simulink model "MCU_FaultDiag"  (R2022b)
settings: Solver=FixedStepDiscrete  StartTime=0.0  StopTime=10.0  FixedStep=1e-4  RelTol=1e-3
values from neighbouring files (symbols this model uses):
  C_Fault_CANFaultAnalogCount_u16 = 0.0    [MCU_FaultDiag_Datadictionary.sldd]    (also in MCU_FaultDiag_Datadictionary_objects.m = myPackage.Parameter)
  C_Fault_CANFaultCoeff_f32 = 0.0    [MCU_FaultDiag_Datadictionary.sldd]    (also in MCU_FaultDiag_Datadictionary_objects.m = myPackage.Parameter)
  C_Fault_CANFaultDiagEn_u8 = 0.0    [MCU_FaultDiag_Datadictionary.sldd]    (also in MCU_FaultDiag_Datadictionary_objects.m = myPackage.Parameter)
  C_Fault_CANFaultErrCode_u16 = 0.0    [MCU_FaultDiag_Datadictionary.sldd]    (also in MCU_FaultDiag_Datadictionary_objects.m = myPackage.Parameter)
  C_Fault_CANFaultLevel_u8 = 0.0    [MCU_FaultDiag_Datadictionary.sldd]    (also in MCU_FaultDiag_Datadictionary_objects.m = myPackage.Parameter)
  C_Fault_CANFaultTestbedCount_u16 = 0.0    [MCU_FaultDiag_Datadictionary.sldd]    (also in MCU_FaultDiag_Datadictionary_objects.m = myPackage.Parameter)
  C_Fault_CANFaultVehicleCount_u16 = 0.0    [MCU_FaultDiag_Datadictionary.sldd]    (also in MCU_FaultDiag_Datadictionary_objects.m = myPackage.Parameter)
  C_Fault_IaCircuitConfirmCnt_u16 = 0.0    [MCU_FaultDiag_Datadictionary.sldd]    (also in MCU_FaultDiag_Datadictionary_objects.m = myPackage.Parameter)
  C_Fault_IaCircuitConfirmDownTh_u16 = 0.0    [MCU_FaultDiag_Datadictionary.sldd]    (also in MCU_FaultDiag_Datadictionary_objects.m = myPackage.Parameter)
  C_Fault_IaCircuitConfirmUpTh_u16 = 0.0    [MCU_FaultDiag_Datadictionary.sldd]    (also in MCU_FaultDiag_Datadictionary_objects.m = myPackage.Parameter)
  C_Fault_IaCircuitFaultCoeff_f32 = 0.0    [MCU_FaultDiag_Datadictionary.sldd]    (also in MCU_FaultDiag_Datadictionary_objects.m = myPackage.Parameter)
  C_Fault_IaCircuitFaultDiagEn_u8 = 0.0    [MCU_FaultDiag_Datadictionary.sldd]    (also in MCU_FaultDiag_Datadictionary_objects.m = myPackage.Parameter)
  C_Fault_IaCircuitFaultLevel_u8 = 0.0    [MCU_FaultDiag_Datadictionary.sldd]    (also in MCU_FaultDiag_Datadictionary_objects.m = myPackage.Parameter)
  C_Fault_IaConfirmCnt_u16 = 0.0    [MCU_FaultDiag_Datadictionary.sldd]    (also in MCU_FaultDiag_Datadictionary_objects.m = myPackage.Parameter; MCU_Fault_Datadictionary_objects.m = myPackage.Parameter; MCU_Fault_Datadictionary_objects.sldd)
  C_Fault_IaInstantFaultCoeff_f32 = 0.0    [MCU_FaultDiag_Datadictionary.sldd]    (also in MCU_FaultDiag_Datadictionary_objects.m = myPackage.Parameter)
  C_Fault_IaInstantFaultDiagEn_u8 = 0.0    [MCU_FaultDiag_Datadictionary.sldd]    (also in MCU_FaultDiag_Datadictionary_objects.m = myPackage.Parameter)
  C_Fault_IaInstantFaultLevel_u8 = 0.0    [MCU_FaultDiag_Datadictionary.sldd]    (also in MCU_FaultDiag_Datadictionary_objects.m = myPackage.Parameter)
  C_Fault_IaOverLoadConfirmCnt_u16 = 0.0    [MCU_FaultDiag_Datadictionary.sldd]    (also in MCU_FaultDiag_Datadictionary_objects.m = myPackage.Parameter)
  C_Fault_IaOverLoadFaultCoeff_f32 = 0.0    [MCU_FaultDiag_Datadictionary.sldd]    (also in MCU_FaultDiag_Datadictionary_objects.m = myPackage.Parameter)
  C_Fault_IaOverLoadFaultDiagEn_u8 = 0.0    [MCU_FaultDiag_Datadictionary.sldd]    (also in MCU_FaultDiag_Datadictionary_objects.m = myPackage.Parameter)
  C_Fault_IaOverLoadFaultErrCode_u16 = 0.0    [MCU_FaultDiag_Datadictionary.sldd]    (also in MCU_FaultDiag_Datadictionary_objects.m = myPackage.Parameter)
  C_Fault_IaOverLoadFaultLevel_u8 = 0.0    [MCU_FaultDiag_Datadictionary.sldd]    (also in MCU_FaultDiag_Datadictionary_objects.m = myPackage.Parameter)
  C_Fault_IbCircuitConfirmCnt_u16 = 0.0    [MCU_FaultDiag_Datadictionary.sldd]    (also in MCU_FaultDiag_Datadictionary_objects.m = myPackage.Parameter)
  C_Fault_IbCircuitConfirmDownTh_u16 = 0.0    [MCU_FaultDiag_Datadictionary.sldd]    (also in MCU_FaultDiag_Datadictionary_objects.m = myPackage.Parameter)
  C_Fault_IbCircuitConfirmUpTh_u16 = 0.0    [MCU_FaultDiag_Datadictionary.sldd]    (also in MCU_FaultDiag_Datadictionary_objects.m = myPackage.Parameter)
  C_Fault_IbCircuitFaultCoeff_f32 = 0.0    [MCU_FaultDiag_Datadictionary.sldd]    (also in MCU_FaultDiag_Datadictionary_objects.m = myPackage.Parameter)
  C_Fault_IbCircuitFaultDiagEn_u8 = 0.0    [MCU_FaultDiag_Datadictionary.sldd]    (also in MCU_FaultDiag_Datadictionary_objects.m = myPackage.Parameter)
  C_Fault_IbCircuitFaultLevel_u8 = 0.0    [MCU_FaultDiag_Datadictionary.sldd]    (also in MCU_FaultDiag_Datadictionary_objects.m = myPackage.Parameter)
  C_Fault_IbConfirmCnt_u16 = 0.0    [MCU_FaultDiag_Datadictionary.sldd]    (also in MCU_FaultDiag_Datadictionary_objects.m = myPackage.Parameter; MCU_Fault_Datadictionary_objects.m = myPackage.Parameter; MCU_Fault_Datadictionary_objects.sldd)
  C_Fault_IbInstantFaultCoeff_f32 = 0.0    [MCU_FaultDiag_Datadictionary.sldd]    (also in MCU_FaultDiag_Datadictionary_objects.m = myPackage.Parameter)
  C_Fault_IbInstantFaultDiagEn_u8 = 0.0    [MCU_FaultDiag_Datadictionary.sldd]    (also in MCU_FaultDiag_Datadictionary_objects.m = myPackage.Parameter)
  C_Fault_IbInstantFaultLevel_u8 = 0.0    [MCU_FaultDiag_Datadictionary.sldd]    (also in MCU_FaultDiag_Datadictionary_objects.m = myPackage.Parameter)
  C_Fault_IbOverLoadConfirmCnt_u16 = 0.0    [MCU_FaultDiag_Datadictionary.sldd]    (also in MCU_FaultDiag_Datadictionary_objects.m = myPackage.Parameter)
  C_Fault_IbOverLoadFaultCoeff_f32 = 0.0    [MCU_FaultDiag_Datadictionary.sldd]    (also in MCU_FaultDiag_Datadictionary_objects.m = myPackage.Parameter)
  C_Fault_IbOverLoadFaultDiagEn_u8 = 0.0    [MCU_FaultDiag_Datadictionary.sldd]    (also in MCU_FaultDiag_Datadictionary_objects.m = myPackage.Parameter)
  C_Fault_IbOverLoadFaultErrCode_u16 = 0.0    [MCU_FaultDiag_Datadictionary.sldd]    (also in MCU_FaultDiag_Datadictionary_objects.m = myPackage.Parameter)
  C_Fault_IbOverLoadFaultLevel_u8 = 0.0    [MCU_FaultDiag_Datadictionary.sldd]    (also in MCU_FaultDiag_Datadictionary_objects.m = myPackage.Parameter)
  C_Fault_IcCircuitConfirmCnt_u16 = 0.0    [MCU_FaultDiag_Datadictionary.sldd]    (also in MCU_FaultDiag_Datadictionary_objects.m = myPackage.Parameter)
  C_Fault_IcCircuitConfirmDownTh_u16 = 0.0    [MCU_FaultDiag_Datadictionary.sldd]    (also in MCU_FaultDiag_Datadictionary_objects.m = myPackage.Parameter)
  C_Fault_IcCircuitConfirmUpTh_u16 = 0.0    [MCU_FaultDiag_Datadictionary.sldd]    (also in MCU_FaultDiag_Datadictionary_objects.m = myPackage.Parameter)
  C_Fault_IcCircuitFaultCoeff_f32 = 0.0    [MCU_FaultDiag_Datadictionary.sldd]    (also in MCU_FaultDiag_Datadictionary_objects.m = myPackage.Parameter)
  C_Fault_IcCircuitFaultDiagEn_u8 = 0.0    [MCU_FaultDiag_Datadictionary.sldd]    (also in MCU_FaultDiag_Datadictionary_objects.m = myPackage.Parameter)
  C_Fault_IcCircuitFaultLevel_u8 = 0.0    [MCU_FaultDiag_Datadictionary.sldd]    (also in MCU_FaultDiag_Datadictionary_objects.m = myPackage.Parameter)
  C_Fault_IcConfirmCnt_u16 = 0.0    [MCU_FaultDiag_Datadictionary.sldd]    (also in MCU_FaultDiag_Datadictionary_objects.m = myPackage.Parameter; MCU_Fault_Datadictionary_objects.m = myPackage.Parameter; MCU_Fault_Datadictionary_objects.sldd)
  C_Fault_IcInstantFaultCoeff_f32 = 0.0    [MCU_FaultDiag_Datadictionary.sldd]    (also in MCU_FaultDiag_Datadictionary_objects.m = myPackage.Parameter)
  C_Fault_IcInstantFaultDiagEn_u8 = 0.0    [MCU_FaultDiag_Datadictionary.sldd]    (also in MCU_FaultDiag_Datadictionary_objects.m = myPackage.Parameter)
  C_Fault_IcInstantFaultLevel_u8 = 0.0    [MCU_FaultDiag_Datadictionary.sldd]    (also in MCU_FaultDiag_Datadictionary_objects.m = myPackage.Parameter)
  C_Fault_IcOverLoadConfirmCnt_u16 = 0.0    [MCU_FaultDiag_Datadictionary.sldd]    (also in MCU_FaultDiag_Datadictionary_objects.m = myPackage.Parameter)
  C_Fault_IcOverLoadFaultCoeff_f32 = 0.0    [MCU_FaultDiag_Datadictionary.sldd]    (also in MCU_FaultDiag_Datadictionary_objects.m = myPackage.Parameter)
  C_Fault_IcOverLoadFaultDiagEn_u8 = 0.0    [MCU_FaultDiag_Datadictionary.sldd]    (also in MCU_FaultDiag_Datadictionary_objects.m = myPackage.Parameter)
  C_Fault_IcOverLoadFaultErrCode_u16 = 0.0    [MCU_FaultDiag_Datadictionary.sldd]    (also in MCU_FaultDiag_Datadictionary_objects.m = myPackage.Parameter)
  C_Fault_IcOverLoadFaultLevel_u8 = 0.0    [MCU_FaultDiag_Datadictionary.sldd]    (also in MCU_FaultDiag_Datadictionary_objects.m = myPackage.Parameter)
  C_Fault_IdcCircuitConfirmCnt_u16 = 0.0    [MCU_FaultDiag_Datadictionary.sldd]    (also in MCU_FaultDiag_Datadictionary_objects.m = myPackage.Parameter)
  C_Fault_IdcCircuitConfirmDownTh_u16 = 0.0    [MCU_FaultDiag_Datadictionary.sldd]    (also in MCU_FaultDiag_Datadictionary_objects.m = myPackage.Parameter)
  C_Fault_IdcCircuitConfirmUpTh_u16 = 0.0    [MCU_FaultDiag_Datadictionary.sldd]    (also in MCU_FaultDiag_Datadictionary_objects.m = myPackage.Parameter)
  C_Fault_IdcCircuitFaultCoeff_f32 = 0.0    [MCU_FaultDiag_Datadictionary.sldd]    (also in MCU_FaultDiag_Datadictionary_objects.m = myPackage.Parameter)
  C_Fault_IdcCircuitFaultDiagEn_u8 = 0.0    [MCU_FaultDiag_Datadictionary.sldd]    (also in MCU_FaultDiag_Datadictionary_objects.m = myPackage.Parameter)
  C_Fault_IdcCircuitFaultLevel_u8 = 0.0    [MCU_FaultDiag_Datadictionary.sldd]    (also in MCU_FaultDiag_Datadictionary_objects.m = myPackage.Parameter)
  C_Fault_SelfCheckFaultCoeff_f32 = 0.0    [MCU_FaultDiag_Datadictionary.sldd]    (also in MCU_FaultDiag_Datadictionary_objects.m = myPackage.Parameter)
  C_Fault_SelfCheckFaultDiagEn_u8 = 0.0    [MCU_FaultDiag_Datadictionary.sldd]    (also in MCU_FaultDiag_Datadictionary_objects.m = myPackage.Parameter)
  C_Fault_SelfCheckFaultLevel_u8 = 0.0    [MCU_FaultDiag_Datadictionary.sldd]    (also in MCU_FaultDiag_Datadictionary_objects.m = myPackage.Parameter)
  C_Fault_SpeedOverConfirmCnt_u16 = 0.0    [MCU_FaultDiag_Datadictionary.sldd]    (also in MCU_FaultDiag_Datadictionary_objects.m = myPackage.Parameter)
  C_Fault_SpeedOverFaultCoeff_f32 = 0.0    [MCU_FaultDiag_Datadictionary.sldd]    (also in MCU_FaultDiag_Datadictionary_objects.m = myPackage.Parameter)
  C_Fault_SpeedOverFaultDiagEn_u8 = 0.0    [MCU_FaultDiag_Datadictionary.sldd]    (also in MCU_FaultDiag_Datadictionary_objects.m = myPackage.Parameter)
  C_Fault_SpeedOverFaultLevel_u8 = 0.0    [MCU_FaultDiag_Datadictionary.sldd]    (also in MCU_FaultDiag_Datadictionary_objects.m = myPackage.Parameter)
  C_Fault_SpeedOverWarnConfirmCnt_u16 = 0.0    [MCU_FaultDiag_Datadictionary.sldd]    (also in MCU_FaultDiag_Datadictionary_objects.m = myPackage.Parameter)
  C_Fault_SpeedOverWarnFaultCoeff_f32 = 0.0    [MCU_FaultDiag_Datadictionary.sldd]    (also in MCU_FaultDiag_Datadictionary_objects.m = myPackage.Parameter)
  C_Fault_SpeedOverWarnFaultDiagEn_u8 = 0.0    [MCU_FaultDiag_Datadictionary.sldd]    (also in MCU_FaultDiag_Datadictionary_objects.m = myPackage.Parameter)
  C_Fault_SpeedOverWarnFaultLevel_u8 = 0.0    [MCU_FaultDiag_Datadictionary.sldd]    (also in MCU_FaultDiag_Datadictionary_objects.m = myPackage.Parameter)
  C_Fault_TigbtCircuitConfirmCnt_u16 = 0.0    [MCU_FaultDiag_Datadictionary.sldd]    (also in MCU_FaultDiag_Datadictionary_objects.m = myPackage.Parameter)
  C_Fault_TigbtCircuitConfirmTh_u16 = 0.0    [MCU_FaultDiag_Datadictionary.sldd]    (also in MCU_FaultDiag_Datadictionary_objects.m = myPackage.Parameter)
  C_Fault_TigbtCircuitFaultCoeff_f32 = 0.0    [MCU_FaultDiag_Datadictionary.sldd]    (also in MCU_FaultDiag_Datadictionary_objects.m = myPackage.Parameter)
  C_Fault_TigbtCircuitFaultDiagEn_u8 = 0.0    [MCU_FaultDiag_Datadictionary.sldd]    (also in MCU_FaultDiag_Datadictionary_objects.m = myPackage.Parameter)
  C_Fault_TigbtCircuitFaultErrCode_u16 = 0.0    [MCU_FaultDiag_Datadictionary.sldd]    (also in MCU_FaultDiag_Datadictionary_objects.m = myPackage.Parameter)
  C_Fault_TigbtCircuitFaultLevel_u8 = 0.0    [MCU_FaultDiag_Datadictionary.sldd]    (also in MCU_FaultDiag_Datadictionary_objects.m = myPackage.Parameter)
  C_Fault_TigbtOverConfirmCnt_u16 = 0.0    [MCU_FaultDiag_Datadictionary.sldd]    (also in MCU_FaultDiag_Datadictionary_objects.m = myPackage.Parameter; MCU_Fault_Datadictionary_objects.m = myPackage.Parameter; MCU_Fault_Datadictionary_objects.sldd)
  C_Fault_TigbtOverFaultCoeff_f32 = 0.0    [MCU_FaultDiag_Datadictionary.sldd]    (also in MCU_FaultDiag_Datadictionary_objects.m = myPackage.Parameter)
  C_Fault_TigbtOverFaultDiagEn_u8 = 0.0    [MCU_FaultDiag_Datadictionary.sldd]    (also in MCU_FaultDiag_Datadictionary_objects.m = myPackage.Parameter)
  C_Fault_TigbtOverFaultLevel_u8 = 0.0    [MCU_FaultDiag_Datadictionary.sldd]    (also in MCU_FaultDiag_Datadictionary_objects.m = myPackage.Parameter)
  C_Fault_TigbtOverWarnConfirmCnt_u16 = 0.0    [MCU_FaultDiag_Datadictionary.sldd]    (also in MCU_FaultDiag_Datadictionary_objects.m = myPackage.Parameter)
  C_Fault_TigbtOverWarnFaultCoeff_f32 = 0.0    [MCU_FaultDiag_Datadictionary.sldd]    (also in MCU_FaultDiag_Datadictionary_objects.m = myPackage.Parameter)
  C_Fault_TigbtOverWarnFaultDiagEn_u8 = 0.0    [MCU_FaultDiag_Datadictionary.sldd]    (also in MCU_FaultDiag_Datadictionary_objects.m = myPackage.Parameter)
  C_Fault_TigbtOverWarnFaultLevel_u8 = 0.0    [MCU_FaultDiag_Datadictionary.sldd]    (also in MCU_FaultDiag_Datadictionary_objects.m = myPackage.Parameter)
  C_Fault_TmotorCircuitConfirmCnt_u16 = 0.0    [MCU_FaultDiag_Datadictionary.sldd]    (also in MCU_FaultDiag_Datadictionary_objects.m = myPackage.Parameter)
  C_Fault_TmotorCircuitConfirmTh_u16 = 0.0    [MCU_FaultDiag_Datadictionary.sldd]    (also in MCU_FaultDiag_Datadictionary_objects.m = myPackage.Parameter)
  C_Fault_TmotorCircuitFaultCoeff_f32 = 0.0    [MCU_FaultDiag_Datadictionary.sldd]    (also in MCU_FaultDiag_Datadictionary_objects.m = myPackage.Parameter)
  C_Fault_TmotorCircuitFaultDiagEn_u8 = 0.0    [MCU_FaultDiag_Datadictionary.sldd]    (also in MCU_FaultDiag_Datadictionary_objects.m = myPackage.Parameter)
  C_Fault_TmotorCircuitFaultErrCode_u16 = 0.0    [MCU_FaultDiag_Datadictionary.sldd]    (also in MCU_FaultDiag_Datadictionary_objects.m = myPackage.Parameter)
  C_Fault_TmotorCircuitFaultLevel_u8 = 0.0    [MCU_FaultDiag_Datadictionary.sldd]    (also in MCU_FaultDiag_Datadictionary_objects.m = myPackage.Parameter)
  C_Fault_TmotorOverConfirmCnt_u16 = 0.0    [MCU_FaultDiag_Datadictionary.sldd]    (also in MCU_FaultDiag_Datadictionary_objects.m = myPackage.Parameter; MCU_Fault_Datadictionary_objects.m = myPackage.Parameter; MCU_Fault_Datadictionary_objects.sldd)
  C_Fault_TmotorOverFaultCoeff_f32 = 0.0    [MCU_FaultDiag_Datadictionary.sldd]    (also in MCU_FaultDiag_Datadictionary_objects.m = myPackage.Parameter)
  C_Fault_TmotorOverFaultDiagEn_u8 = 0.0    [MCU_FaultDiag_Datadictionary.sldd]    (also in MCU_FaultDiag_Datadictionary_objects.m = myPackage.Parameter)
  C_Fault_TmotorOverFaultLevel_u8 = 0.0    [MCU_FaultDiag_Datadictionary.sldd]    (also in MCU_FaultDiag_Datadictionary_objects.m = myPackage.Parameter)
  C_Fault_TmotorOverWarnConfirmCnt_u16 = 0.0    [MCU_FaultDiag_Datadictionary.sldd]    (also in MCU_FaultDiag_Datadictionary_objects.m = myPackage.Parameter)
  C_Fault_TmotorOverWarnFaultCoeff_f32 = 0.0    [MCU_FaultDiag_Datadictionary.sldd]    (also in MCU_FaultDiag_Datadictionary_objects.m = myPackage.Parameter)
  C_Fault_TmotorOverWarnFaultDiagEn_u8 = 0.0    [MCU_FaultDiag_Datadictionary.sldd]    (also in MCU_FaultDiag_Datadictionary_objects.m = myPackage.Parameter)
  C_Fault_TmotorOverWarnFaultLevel_u8 = 0.0    [MCU_FaultDiag_Datadictionary.sldd]    (also in MCU_FaultDiag_Datadictionary_objects.m = myPackage.Parameter)
  C_Fault_TpcuCircuitConfirmCnt_u16 = 0.0    [MCU_FaultDiag_Datadictionary.sldd]    (also in MCU_FaultDiag_Datadictionary_objects.m = myPackage.Parameter)
  C_Fault_TpcuCircuitConfirmTh_u16 = 0.0    [MCU_FaultDiag_Datadictionary.sldd]    (also in MCU_FaultDiag_Datadictionary_objects.m = myPackage.Parameter)
  C_Fault_TpcuCircuitFaultCoeff_f32 = 0.0    [MCU_FaultDiag_Datadictionary.sldd]    (also in MCU_FaultDiag_Datadictionary_objects.m = myPackage.Parameter)
  C_Fault_TpcuCircuitFaultDiagEn_u8 = 0.0    [MCU_FaultDiag_Datadictionary.sldd]    (also in MCU_FaultDiag_Datadictionary_objects.m = myPackage.Parameter)
  C_Fault_TpcuCircuitFaultErrCode_u16 = 0.0    [MCU_FaultDiag_Datadictionary.sldd]    (also in MCU_FaultDiag_Datadictionary_objects.m = myPackage.Parameter)
  C_Fault_TpcuCircuitFaultLevel_u8 = 0.0    [MCU_FaultDiag_Datadictionary.sldd]    (also in MCU_FaultDiag_Datadictionary_objects.m = myPackage.Parameter)
  C_Fault_TZFaultCoeff_f32 = 0.0    [MCU_FaultDiag_Datadictionary.sldd]    (also in MCU_FaultDiag_Datadictionary_objects.m = myPackage.Parameter)
  C_Fault_TZFaultDiagEn_u8 = 0.0    [MCU_FaultDiag_Datadictionary.sldd]    (also in MCU_FaultDiag_Datadictionary_objects.m = myPackage.Parameter)
  C_Fault_TZFaultLevel_u8 = 0.0    [MCU_FaultDiag_Datadictionary.sldd]    (also in MCU_FaultDiag_Datadictionary_objects.m = myPackage.Parameter)
  C_Fault_UdcCircuitConfirmCnt_u16 = 0.0    [MCU_FaultDiag_Datadictionary.sldd]    (also in MCU_FaultDiag_Datadictionary_objects.m = myPackage.Parameter)
  C_Fault_UdcCircuitConfirmTh_u16 = 0.0    [MCU_FaultDiag_Datadictionary.sldd]    (also in MCU_FaultDiag_Datadictionary_objects.m = myPackage.Parameter)
  C_Fault_UdcCircuitFaultCoeff_f32 = 0.0    [MCU_FaultDiag_Datadictionary.sldd]    (also in MCU_FaultDiag_Datadictionary_objects.m = myPackage.Parameter)
  C_Fault_UdcCircuitFaultDiagEn_u8 = 0.0    [MCU_FaultDiag_Datadictionary.sldd]    (also in MCU_FaultDiag_Datadictionary_objects.m = myPackage.Parameter)
  C_Fault_UdcCircuitFaultErrCode_u16 = 0.0    [MCU_FaultDiag_Datadictionary.sldd]    (also in MCU_FaultDiag_Datadictionary_objects.m = myPackage.Parameter)
  C_Fault_UdcCircuitFaultLevel_u8 = 0.0    [MCU_FaultDiag_Datadictionary.sldd]    (also in MCU_FaultDiag_Datadictionary_objects.m = myPackage.Parameter)
  C_Fault_UdcOverConfirmCnt_u16 = 0.0    [MCU_FaultDiag_Datadictionary.sldd]    (also in MCU_FaultDiag_Datadictionary_objects.m = myPackage.Parameter)
  C_Fault_UdcOverFaultCoeff_f32 = 0.0    [MCU_FaultDiag_Datadictionary.sldd]    (also in MCU_FaultDiag_Datadictionary_objects.m = myPackage.Parameter)
  C_Fault_UdcOverFaultDiagEn_u8 = 0.0    [MCU_FaultDiag_Datadictionary.sldd]    (also in MCU_FaultDiag_Datadictionary_objects.m = myPackage.Parameter)
  C_Fault_UdcOverFaultLevel_u8 = 0.0    [MCU_FaultDiag_Datadictionary.sldd]    (also in MCU_FaultDiag_Datadictionary_objects.m = myPackage.Parameter)
  C_Fault_UdcOverWarnConfirmCnt_u16 = 0.0    [MCU_FaultDiag_Datadictionary.sldd]    (also in MCU_FaultDiag_Datadictionary_objects.m = myPackage.Parameter)
  C_Fault_UdcOverWarnFaultCoeff_f32 = 0.0    [MCU_FaultDiag_Datadictionary.sldd]    (also in MCU_FaultDiag_Datadictionary_objects.m = myPackage.Parameter)
  C_Fault_UdcOverWarnFaultDiagEn_u8 = 0.0    [MCU_FaultDiag_Datadictionary.sldd]    (also in MCU_FaultDiag_Datadictionary_objects.m = myPackage.Parameter)
  C_Fault_UdcOverWarnFaultLevel_u8 = 0.0    [MCU_FaultDiag_Datadictionary.sldd]    (also in MCU_FaultDiag_Datadictionary_objects.m = myPackage.Parameter)
  ... (+8 more)
undefined symbols (not defined in the file or in its folder): AB_SAMPLE, ABC_SAMPLE, AC_SAMPLE, cAgeingMode, cSingleBoardMode, ParamCfg_CommandSource_u16, ParamCfg_IaValueDefault_u16, ParamCfg_IbValueDefault_u16, ParamCfg_IcValueDefault_u16, ParamCfg_IphaseLimitStart_u16, ParamCfg_MotorLimitStart_u16, ParamCfg_MotorLimitStop_u16, ParamCfg_SampleMode_u16, ParamCfg_SpeedLimitStart_u16, ParamCfg_SpeedLimitStop_u16, ParamCfg_TigbtLimitStart_u16, ParamCfg_TigbtLimitStop_u16, VEHICLE
libraries: simulink x62
(part 1 of 426)
settings Model: DataDictionary=MCU_FaultDiag_Datadictionary.sldd  Creator=ZYH  LastModifiedBy=ZYH
settings OptimizationCC: DefaultParameterBehavior=Inlined  EnhancedBackFolding=on  PassReuseOutputArgsAs=Individual arguments  OptimizeBlockOrder=speed  DifferentSizesBufferReuse=on  OptimizationCustomize=off  EfficientTunableParamExpr=on
settings DebuggingCC: ParameterTunabilityLossMsg=error
settings SFSimCC: MATLABDynamicMemAlloc=off
settings RTWCC: Description=Embedded Coder  SystemTargetFile=ert.tlc  GenCodeOnly=on  TemplateMakefile=ert_default_tmf
settings CodeAppCC: ForceParamTrailComments=on  IgnoreCustomStorageClasses=off  OperatorAnnotations=on  SimulinkDataObjDesc=on  SFDataObjDesc=on  InsertBlockDesc=on
settings ERTTargetCC: TargetLangStandard=C99 (ISO)  GenerateSampleERTMain=on  InlinedParameterPlacement=NonHierarchical  ERTCustomFileTemplate=example_file_process.tlc

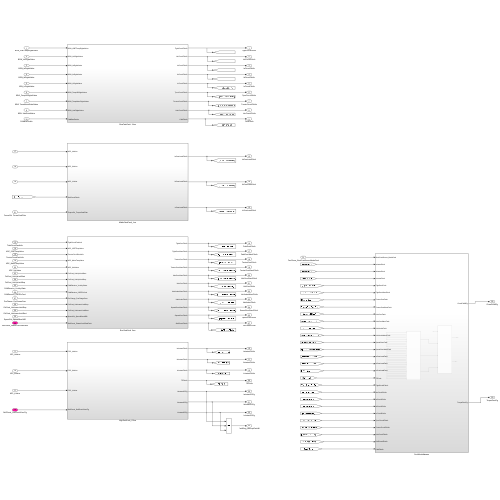
[thumbnail: Simulink's stored preview of the top-level diagram]
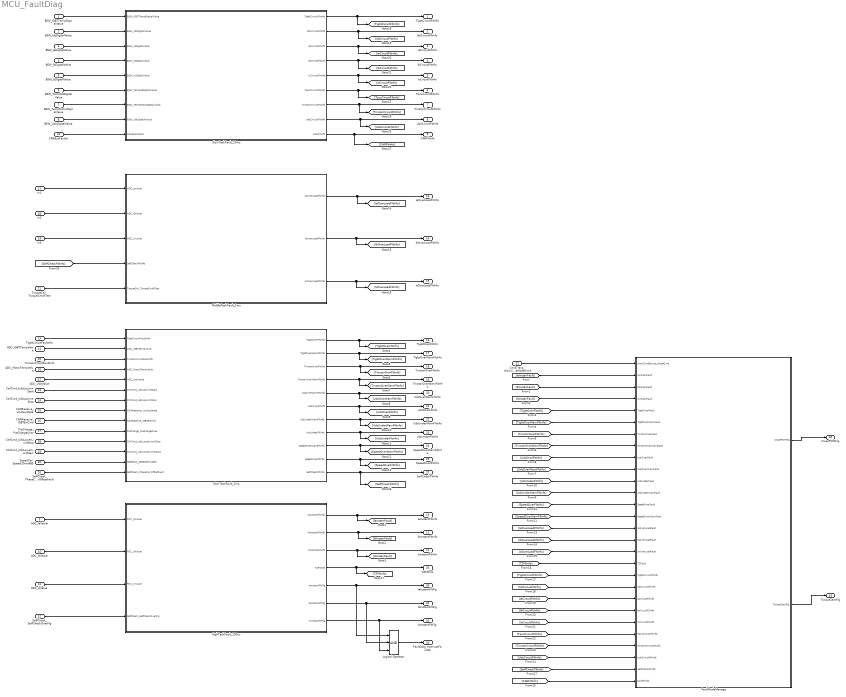
== system MCU_FaultDiag ==
  BSW_IGBTTempDigitalValue : Inport
  BSW_IdcDigitalValue : Inport  Port=2
  BSW_IaDigitalValue : Inport  Port=3
  BSW_IbDigitalValue : Inport  Port=4
  BSW_IcDigitalValue : Inport  Port=5
  BSW_TempHSDigitalValue : Inport  Port=6
  BSW_TempMotorDigitalValue : Inport  Port=7
  BSW_UdcDigitalValue : Inport  Port=8
  ADC_IaValue : Inport  Port=9
  ADC_IbValue : Inport  Port=10
  ADC_IcValue : Inport  Port=11
  SelfCheck_SelfCheckOverFlg : Inport  Port=12
  TigbtCircuitFaultInfo : Inport  Port=13  OutDataTypeStr=Bus: FaultBus
  ADC_IGBTTempValue : Inport  Port=14
  TmotorCircuitFaultInfo : Inport  Port=15  OutDataTypeStr=Bus: FaultBus
  ADC_MotorTempValue : Inport  Port=16
  In1 : Inport  Port=17
  In2 : Inport  Port=18
  In3 : Inport  Port=19
  SelfCheck_PhaseCurrOffsetFault : Inport  Port=20
  TorqueCtrl_TorqueCmdFilter : Inport  Port=21
  ADC_UdcValue : Inport  Port=22
  CtrlCmd_UdcUpLimitStart : Inport  Port=23
  CtrlCmd_UdcUpLimitStop : Inport  Port=24
  CANReceive_VcuKeyState : Inport  Port=25
  CANReceive_IGBTEnCmd : Inport  Port=26
  PreCharge_PreChargeOver : Inport  Port=27
  CtrlCmd_UdcLowerLimitStop : Inport  Port=28
  CtrlCmd_UdcLowerLimitStart : Inport  Port=29
  SpeedCal_Speed20msABS : Inport  Port=30
  CmdTrans_WorkCmdSourceModeCmd : Inport  Port=31
  CANBusFaultIn : Inport  Port=32
  FaultModeManage : Subsystem
  HighTaskFault_100us : Subsystem
  Logical Operator : Logic  Inputs=3  AllPortsSameDT=off  OutDataTypeStr=boolean
  MiddleTaskFault_1ms : Subsystem
  SlowTaskFault_10ms : Subsystem
  SlowTaskFault_2ms : Subsystem
  TigbtCircuitFltInfo : Outport
  IdcCircuitFltInfo : Outport  Port=2
  IaCircuitFltInfo : Outport  Port=3
  IbCircuitFltInfo : Outport  Port=4
  IcCircuitFltInfo : Outport  Port=5
  TpcuCircuitFltInfo : Outport  Port=6
  TmotorCircuitFltInfo : Outport  Port=7
  UdcCircuitFltInfo : Outport  Port=8
  CANFltInfo : Outport  Port=9
  IaInstantFltInfo : Outport  Port=10
  IbInstantFltInfo : Outport  Port=11
  IcInstantFltInfo : Outport  Port=12
  IaOverLoadFltInfo : Outport  Port=13
  IbOverLoadFltInfo : Outport  Port=14
  IcOverLoadFltInfo : Outport  Port=15
  TigbtOverFltInfo : Outport  Port=16
  TigbtOverWarnFltInfo : Outport  Port=17
  TmotorOverFltInfo : Outport  Port=18
  TmotorOverWarnFltInfo : Outport  Port=19
  UdcOverWarnFltInfo : Outport  Port=20
  UdcOverFltInfo : Outport  Port=21
  UdcUnderWarnFltInfo : Outport  Port=22
  UdcUnderFltInfo : Outport  Port=23
  SpeedOverWarnFltInfo : Outport  Port=24
  SpeedOverFltInfo : Outport  Port=25
  TZFltInfo : Outport  Port=26
  SelfCheckFltInfo : Outport  Port=27
  ClosePWMFlg : Outport  Port=28
  TorqueZeroFlg : Outport  Port=29
  IaInstantFltFlg : Outport  Port=30
  IbInstantFltFlg : Outport  Port=31
  IcInstantFltFlg : Outport  Port=32
  FaultDiag_InterruptFaultAll : Outport  Port=33
  wires:
  ADC_IaValue/1 -> HighTaskFault_100us/1(FOC_IaValue)
  ADC_IbValue/1 -> HighTaskFault_100us/2(FOC_IbValue)
  ADC_IcValue/1 -> HighTaskFault_100us/3(FOC_IcValue)
  BSW_IGBTTempDigitalValue/1 -> SlowTaskFault_10ms/1(BSW_IGBTTempDigitalValue)
  SlowTaskFault_10ms/1(TigbtCircuitFltInfo) -> [TigbtCircuitFltInfo], TigbtCircuitFltInfo/1
  HighTaskFault_100us/1(IaInstantFltInfo) -> [IaInstanFault], IaInstantFltInfo/1
  HighTaskFault_100us/2(IbInstantFltInfo) -> [IbInstanFault], IbInstantFltInfo/1
  HighTaskFault_100us/3(IcInstantFltInfo) -> [IcInstanFault], IcInstantFltInfo/1
  BSW_IdcDigitalValue/1 -> SlowTaskFault_10ms/2(BSW_IdcDigitalValue)
  BSW_IaDigitalValue/1 -> SlowTaskFault_10ms/3(BSW_IaDigitalValue)
  BSW_IbDigitalValue/1 -> SlowTaskFault_10ms/4(BSW_IbDigitalValue)
  BSW_IcDigitalValue/1 -> SlowTaskFault_10ms/5(BSW_IcDigitalValue)
  SlowTaskFault_10ms/4(IbCircuitFltInfo) -> [IbCircuitFltInfo], IbCircuitFltInfo/1
  SlowTaskFault_10ms/3(IaCircuitFltInfo) -> [IaCircuitFltInfo], IaCircuitFltInfo/1
  SlowTaskFault_10ms/5(IcCircuitFltInfo) -> [IcCircuitFltInfo], IcCircuitFltInfo/1
  SlowTaskFault_10ms/7(TmotorCircuitFltInfo) -> [TmotorCircuitFltInfo], TmotorCircuitFltInfo/1
  SlowTaskFault_10ms/8(UdcCircuitFltInfo) -> [UdcCircuitFltInfo], UdcCircuitFltInfo/1
  BSW_TempHSDigitalValue/1 -> SlowTaskFault_10ms/6(BSW_TempHSDigitalValue)
  BSW_TempMotorDigitalValue/1 -> SlowTaskFault_10ms/7(BSW_TempMotorDigitalValue)
  BSW_UdcDigitalValue/1 -> SlowTaskFault_10ms/8(BSW_UdcDigitalValue)
  TigbtCircuitFaultInfo/1 -> SlowTaskFault_2ms/1(TigbtCircuitFaultInfo)
  TmotorCircuitFaultInfo/1 -> SlowTaskFault_2ms/3(TmotorCircuitFaultInfo)
  ADC_MotorTempValue/1 -> SlowTaskFault_2ms/4(ADC_MotorTempValue)
  ADC_IGBTTempValue/1 -> SlowTaskFault_2ms/2(ADC_IGBTTempValue)
  In1/1 -> MiddleTaskFault_1ms/1(ADC_IaValue)
  In2/1 -> MiddleTaskFault_1ms/2(ADC_IbValue)
  In3/1 -> MiddleTaskFault_1ms/3(ADC_IcValue)
  MiddleTaskFault_1ms/1(IaOverLoadFltInfo) -> IaOverLoadFltInfo/1, [IaOverLoadFltInfo]
  MiddleTaskFault_1ms/2(IbOverLoadFltInfo) -> [IbOverLoadFltInfo], IbOverLoadFltInfo/1
  MiddleTaskFault_1ms/3(IcOverLoadFltInfo) -> [IcOverLoadFltInfo], IcOverLoadFltInfo/1
  TorqueCtrl_TorqueCmdFilter/1 -> MiddleTaskFault_1ms/5(TorqueCtrl_TorqueCmdFilter)
  CtrlCmd_UdcUpLimitStop/1 -> SlowTaskFault_2ms/7(CtrlCmd_UdcUpLimitStop)
  CANReceive_VcuKeyState/1 -> SlowTaskFault_2ms/8(CANReceive_VcuKeyState)
  CANReceive_IGBTEnCmd/1 -> SlowTaskFault_2ms/9(CANReceive_IGBTEnCmd)
  PreCharge_PreChargeOver/1 -> SlowTaskFault_2ms/10(PreCharge_PreChargeOver)
  ADC_UdcValue/1 -> SlowTaskFault_2ms/5(ADC_UdcValue)
  CtrlCmd_UdcLowerLimitStop/1 -> SlowTaskFault_2ms/11(CtrlCmd_UdcLowerLimitStop)
  CtrlCmd_UdcUpLimitStart/1 -> SlowTaskFault_2ms/6(CtrlCmd_UdcUpLimitStart)
  CtrlCmd_UdcLowerLimitStart/1 -> SlowTaskFault_2ms/12(CtrlCmd_UdcLowerLimitStart)
  SpeedCal_Speed20msABS/1 -> SlowTaskFault_2ms/13(SpeedCal_Speed20msABS)
  SlowTaskFault_2ms/1(TigbtOverFltInfo) -> TigbtOverFltInfo/1, [TigbtOverFltInfo]
  SlowTaskFault_2ms/3(TmotorOverFltInfo) -> [TmotorOverFltInfo], TmotorOverFltInfo/1
  SlowTaskFault_2ms/2(TigbtOverWarnFltInfo) -> [TigbtOverWarnFltInfo], TigbtOverWarnFltInfo/1
  SlowTaskFault_2ms/4(TmotorOverWarnFltInfo) -> [TmotorOverWarnFltInfo], TmotorOverWarnFltInfo/1
  SlowTaskFault_2ms/5(UdcOverWarnFltInfo) -> [UdcOverWarnFltInfo], UdcOverWarnFltInfo/1
  SlowTaskFault_2ms/6(UdcOverFltInfo) -> [UdcOverFltInfo], UdcOverFltInfo/1
  SlowTaskFault_2ms/7(UdcUnderWarnFltInfo) -> [UdcUnderWarnFltInfo], UdcUnderWarnFltInfo/1
  SlowTaskFault_2ms/8(UdcUnderFltInfo) -> [UdcUnderFltInfo], UdcUnderFltInfo/1
  SlowTaskFault_2ms/9(SpeedOverWarnFltInfo) -> SpeedOverWarnFltInfo/1, [SpeedOverWarnFltInfo]
  SlowTaskFault_2ms/10(SpeedOverFltInfo) -> [SpeedOverFltInfo], SpeedOverFltInfo/1
  CmdTrans_WorkCmdSourceModeCmd/1 -> FaultModeManage/1(WorkCmdSource_ModeCmd)
  [IaInstanFault] -> FaultModeManage/2(IaInstanFault)
  [IbInstanFault] -> FaultModeManage/3(IbInstanFault)
  [IcInstanFault] -> FaultModeManage/4(IcInstanFault)
  [TigbtOverFltInfo] -> FaultModeManage/5(TigbtOverFault)
  [TigbtOverWarnFltInfo] -> FaultModeManage/6(TigbtOverWarnFault)
  [TmotorOverFltInfo] -> FaultModeManage/7(TmotorOverFault)
  [TmotorOverWarnFltInfo] -> FaultModeManage/8(TmotorOverWarnFault)
  [SpeedOverFltInfo] -> FaultModeManage/13(SpeedOverFault)
  [SpeedOverWarnFltInfo] -> FaultModeManage/14(SpeedOverWarnFault)
  [UdcOverFltInfo] -> FaultModeManage/9(UdcOverFault)
  [UdcOverWarnFltInfo] -> FaultModeManage/10(UdcOverWarnFault)
  [UdcUnderWarnFltInfo] -> FaultModeManage/12(UdcUnderWarnFault)
  [UdcUnderFltInfo] -> FaultModeManage/11(UdcUnderFault)
  [IaOverLoadFltInfo] -> FaultModeManage/15(IaOverLoadFault)
  [IbOverLoadFltInfo] -> FaultModeManage/16(IbOverLoadFault)
  [IcOverLoadFltInfo] -> FaultModeManage/17(IcOverLoadFault)
  HighTaskFault_100us/4(TZFltInfo) -> [TZFltInfo], TZFltInfo/1
  [TZFltInfo] -> FaultModeManage/18(TZFault)
  SlowTaskFault_10ms/2(IdcCircuitFltInfo) -> [IdcCircuitFltInfo], IdcCircuitFltInfo/1
  SlowTaskFault_10ms/6(TpcuCircuitFltInfo) -> [TpcuCircuitFltInfo], TpcuCircuitFltInfo/1
  [TpcuCircuitFltInfo] -> FaultModeManage/24(TpcuCircuitFltInfo)
  [IcCircuitFltInfo] -> FaultModeManage/23(IcCircuitFltInfo)
  [TmotorCircuitFltInfo] -> FaultModeManage/25(TmotorCircuitFltInfo)
  [IbCircuitFltInfo] -> FaultModeManage/22(IbCircuitFltInfo)
  [UdcCircuitFltInfo] -> FaultModeManage/26(UdcCircuitFltInfo)
  [IaCircuitFltInfo] -> FaultModeManage/21(IaCircuitFltInfo)
  [IdcCircuitFltInfo] -> FaultModeManage/20(IdcCircuitFltInfo)
  [TigbtCircuitFltInfo] -> FaultModeManage/19(TigbtCircuitFltInfo)
  [SelfCheckFltInfo] -> FaultModeManage/27(SelfCheckFltInfo)
  SelfCheck_SelfCheckOverFlg/1 -> HighTaskFault_100us/4(SelfCheck_SelfCheckOverFlg)
  SelfCheck_PhaseCurrOffsetFault/1 -> SlowTaskFault_2ms/14(SelfCheck_PhaseCurrOffsetFault)
  SlowTaskFault_2ms/11(SelfCheckFltInfo) -> [SelfCheckFltInfo], SelfCheckFltInfo/1
  [SelfCheckFltInfo] -> MiddleTaskFault_1ms/4(SelfCheckFltInfo)
  FaultModeManage/1(ClosePWMFlg) -> ClosePWMFlg/1
  FaultModeManage/2(TorqueZeroFlg) -> TorqueZeroFlg/1
  HighTaskFault_100us/5(IaInstantFltFlg) -> Logical Operator/1, IaInstantFltFlg/1
  HighTaskFault_100us/6(IbInstantFltFlg) -> Logical Operator/2, IbInstantFltFlg/1
  HighTaskFault_100us/7(IcInstantFltFlg) -> Logical Operator/3, IcInstantFltFlg/1
  Logical Operator/1 -> FaultDiag_InterruptFaultAll/1
  CANBusFaultIn/1 -> SlowTaskFault_10ms/9(CANBusFaultIn)
  SlowTaskFault_10ms/9(CANFltInfo) -> [CANFltInfo], CANFltInfo/1
  [CANFltInfo] -> FaultModeManage/28(CANFltInfo)

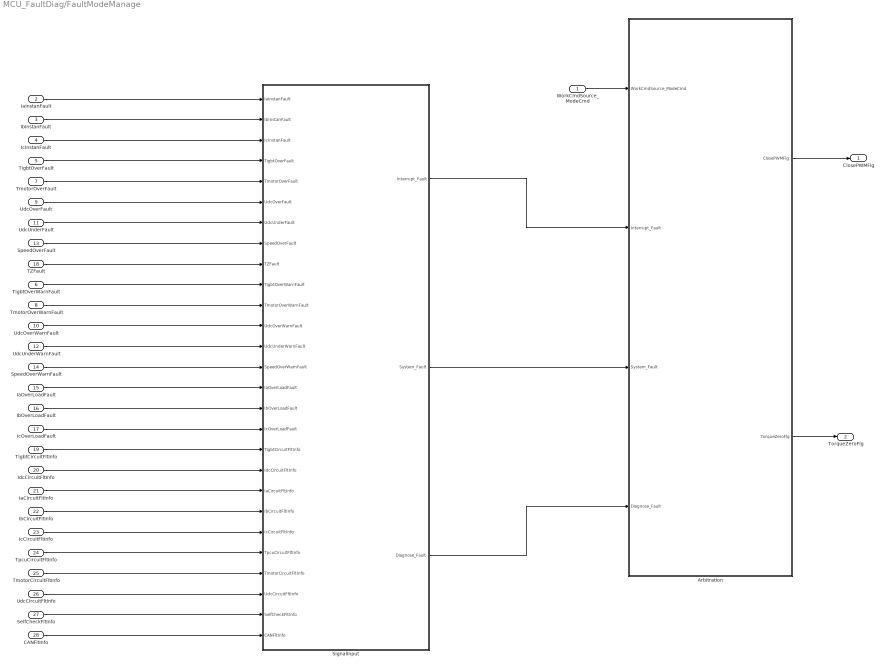
== system MCU_FaultDiag/FaultModeManage ==
  WorkCmdSource_ModeCmd : Inport
  IaInstanFault : Inport  Port=2
  IbInstanFault : Inport  Port=3
  IcInstanFault : Inport  Port=4
  TigbtOverFault : Inport  Port=5
  TigbtOverWarnFault : Inport  Port=6
  TmotorOverFault : Inport  Port=7
  TmotorOverWarnFault : Inport  Port=8
  UdcOverFault : Inport  Port=9
  UdcOverWarnFault : Inport  Port=10
  UdcUnderFault : Inport  Port=11
  UdcUnderWarnFault : Inport  Port=12
  SpeedOverFault : Inport  Port=13
  SpeedOverWarnFault : Inport  Port=14
  IaOverLoadFault : Inport  Port=15
  IbOverLoadFault : Inport  Port=16
  IcOverLoadFault : Inport  Port=17
  TZFault : Inport  Port=18
  TigbtCircuitFltInfo : Inport  Port=19
  IdcCircuitFltInfo : Inport  Port=20
  IaCircuitFltInfo : Inport  Port=21
  IbCircuitFltInfo : Inport  Port=22
  IcCircuitFltInfo : Inport  Port=23
  TpcuCircuitFltInfo : Inport  Port=24
  TmotorCircuitFltInfo : Inport  Port=25
  UdcCircuitFltInfo : Inport  Port=26
  SelfCheckFltInfo : Inport  Port=27
  CANFltInfo : Inport  Port=28
  Arbitration : Subsystem
  SignalInput : Subsystem
  ClosePWMFlg : Outport
  TorqueZeroFlg : Outport  Port=2
  wires:
  IaInstanFault/1 -> SignalInput/1(IaInstanFault)
  IbInstanFault/1 -> SignalInput/2(IbInstanFault)
  IcInstanFault/1 -> SignalInput/3(IcInstanFault)
  TigbtOverFault/1 -> SignalInput/4(TigbtOverFault)
  TmotorOverFault/1 -> SignalInput/5(TmotorOverFault)
  UdcOverFault/1 -> SignalInput/6(UdcOverFault)
  UdcUnderFault/1 -> SignalInput/7(UdcUnderFault)
  SpeedOverFault/1 -> SignalInput/8(SpeedOverFault)
  TZFault/1 -> SignalInput/9(TZFault)
  TigbtOverWarnFault/1 -> SignalInput/10(TigbtOverWarnFault)
  TmotorOverWarnFault/1 -> SignalInput/11(TmotorOverWarnFault)
  UdcOverWarnFault/1 -> SignalInput/12(UdcOverWarnFault)
  UdcUnderWarnFault/1 -> SignalInput/13(UdcUnderWarnFault)
  SpeedOverWarnFault/1 -> SignalInput/14(SpeedOverWarnFault)
  IaOverLoadFault/1 -> SignalInput/15(IaOverLoadFault)
  IbOverLoadFault/1 -> SignalInput/16(IbOverLoadFault)
  IcOverLoadFault/1 -> SignalInput/17(IcOverLoadFault)
  TigbtCircuitFltInfo/1 -> SignalInput/18(TigbtCircuitFltInfo)
  IdcCircuitFltInfo/1 -> SignalInput/19(IdcCircuitFltInfo)
  IaCircuitFltInfo/1 -> SignalInput/20(IaCircuitFltInfo)
  IbCircuitFltInfo/1 -> SignalInput/21(IbCircuitFltInfo)
  IcCircuitFltInfo/1 -> SignalInput/22(IcCircuitFltInfo)
  TpcuCircuitFltInfo/1 -> SignalInput/23(TpcuCircuitFltInfo)
  TmotorCircuitFltInfo/1 -> SignalInput/24(TmotorCircuitFltInfo)
  UdcCircuitFltInfo/1 -> SignalInput/25(UdcCircuitFltInfo)
  SelfCheckFltInfo/1 -> SignalInput/26(SelfCheckFltInfo)
  SignalInput/1(Interrupt_Fault) -> Arbitration/2(Interrupt_Fault)
  WorkCmdSource_ModeCmd/1 -> Arbitration/1(WorkCmdSource_ModeCmd)
  SignalInput/2(System_Fault) -> Arbitration/3(System_Fault)
  SignalInput/3(Diagnose_Fault) -> Arbitration/4(Diagnose_Fault)
  Arbitration/1(ClosePWMFlg) -> ClosePWMFlg/1
  Arbitration/2(TorqueZeroFlg) -> TorqueZeroFlg/1
  CANFltInfo/1 -> SignalInput/27(CANFltInfo)

== system MCU_FaultDiag/HighTaskFault_100us ==
  FOC_IaValue : Inport
  FOC_IbValue : Inport  Port=2
  FOC_IcValue : Inport  Port=3
  SelfCheck_SelfCheckOverFlg : Inport  Port=4
  Bus Selector : BusSelector  OutputSignals=IaInstantFltFlg
  Bus Selector1 : BusSelector  OutputSignals=IbInstantFltFlg
  Bus Selector2 : BusSelector  OutputSignals=IcInstantFltCoeff
  InterruptFaultCheck_100us : Subsystem  TreatAsAtomicUnit=on
      settings: RTWSystemCode=Nonreusable function
  IaInstantFltInfo : Outport
  IbInstantFltInfo : Outport  Port=2
  IcInstantFltInfo : Outport  Port=3
  TZFltInfo : Outport  Port=4
  IaInstantFltFlg : Outport  Port=5
  IbInstantFltFlg : Outport  Port=6
  IcInstantFltFlg : Outport  Port=7
  wires:
  FOC_IcValue/1 -> InterruptFaultCheck_100us/3(FOC_IcValue)
  FOC_IbValue/1 -> InterruptFaultCheck_100us/2(FOC_IbValue)
  FOC_IaValue/1 -> InterruptFaultCheck_100us/1(FOC_IaValue)
  InterruptFaultCheck_100us/1(IaInstantFltInfo) -> Bus Selector/1, IaInstantFltInfo/1
  InterruptFaultCheck_100us/2(IbInstantFltInfo) -> Bus Selector1/1, IbInstantFltInfo/1
  InterruptFaultCheck_100us/3(IcInstantFltInfo) -> Bus Selector2/1, IcInstantFltInfo/1
  SelfCheck_SelfCheckOverFlg/1 -> InterruptFaultCheck_100us/4(SelfCheck_SelfCheckOverFlg)
  InterruptFaultCheck_100us/4(TZFltInfo) -> TZFltInfo/1
  Bus Selector/1 -> IaInstantFltFlg/1  "<IaInstantFltFlg>"
  Bus Selector1/1 -> IbInstantFltFlg/1  "<IbInstantFltFlg>"
  Bus Selector2/1 -> IcInstantFltFlg/1  "<IcInstantFltCoeff>"

== system MCU_FaultDiag/MiddleTaskFault_1ms ==
  note: System_Warn
  ADC_IaValue : Inport
  ADC_IbValue : Inport  Port=2
  ADC_IcValue : Inport  Port=3
  SelfCheckFltInfo : Inport  Port=4
  TorqueCtrl_TorqueCmdFilter : Inport  Port=5
  PhaseFaultCheck : Subsystem
  IaOverLoadFltInfo : Outport
  IbOverLoadFltInfo : Outport  Port=2
  IcOverLoadFltInfo : Outport  Port=3
  wires:
  ADC_IaValue/1 -> PhaseFaultCheck/1(ADC_IaValue)
  ADC_IbValue/1 -> PhaseFaultCheck/3(ADC_IbValue)
  ADC_IcValue/1 -> PhaseFaultCheck/4(ADC_IcValue)
  SelfCheckFltInfo/1 -> PhaseFaultCheck/2(SelfCheckFltInfo)
  TorqueCtrl_TorqueCmdFilter/1 -> PhaseFaultCheck/5(TorqueCtrl_TorqueCmdFilter)
  PhaseFaultCheck/3(IcOverLoadFltInfo) -> IcOverLoadFltInfo/1
  PhaseFaultCheck/2(IbOverLoadFltInfo) -> IbOverLoadFltInfo/1
  PhaseFaultCheck/1(IaOverLoadFltInfo) -> IaOverLoadFltInfo/1

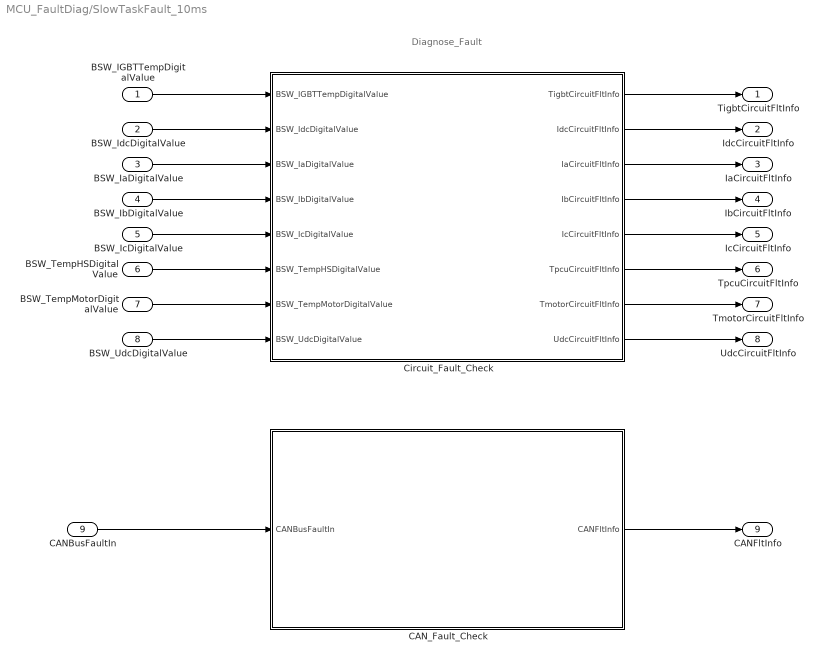
== system MCU_FaultDiag/SlowTaskFault_10ms ==
  note: Diagnose_Fault
  BSW_IGBTTempDigitalValue : Inport
  BSW_IdcDigitalValue : Inport  Port=2
  BSW_IaDigitalValue : Inport  Port=3
  BSW_IbDigitalValue : Inport  Port=4
  BSW_IcDigitalValue : Inport  Port=5
  BSW_TempHSDigitalValue : Inport  Port=6
  BSW_TempMotorDigitalValue : Inport  Port=7
  BSW_UdcDigitalValue : Inport  Port=8
  CANBusFaultIn : Inport  Port=9
  CAN_Fault_Check : Subsystem
  Circuit_Fault_Check : Subsystem
  TigbtCircuitFltInfo : Outport
  IdcCircuitFltInfo : Outport  Port=2
  IaCircuitFltInfo : Outport  Port=3
  IbCircuitFltInfo : Outport  Port=4
  IcCircuitFltInfo : Outport  Port=5
  TpcuCircuitFltInfo : Outport  Port=6
  TmotorCircuitFltInfo : Outport  Port=7
  UdcCircuitFltInfo : Outport  Port=8
  CANFltInfo : Outport  Port=9
  wires:
  BSW_IGBTTempDigitalValue/1 -> Circuit_Fault_Check/1(BSW_IGBTTempDigitalValue)
  Circuit_Fault_Check/1(TigbtCircuitFltInfo) -> TigbtCircuitFltInfo/1
  BSW_IdcDigitalValue/1 -> Circuit_Fault_Check/2(BSW_IdcDigitalValue)
  Circuit_Fault_Check/2(IdcCircuitFltInfo) -> IdcCircuitFltInfo/1
  BSW_IbDigitalValue/1 -> Circuit_Fault_Check/4(BSW_IbDigitalValue)
  BSW_IcDigitalValue/1 -> Circuit_Fault_Check/5(BSW_IcDigitalValue)
  BSW_IaDigitalValue/1 -> Circuit_Fault_Check/3(BSW_IaDigitalValue)
  Circuit_Fault_Check/5(IcCircuitFltInfo) -> IcCircuitFltInfo/1
  Circuit_Fault_Check/4(IbCircuitFltInfo) -> IbCircuitFltInfo/1
  Circuit_Fault_Check/3(IaCircuitFltInfo) -> IaCircuitFltInfo/1
  BSW_UdcDigitalValue/1 -> Circuit_Fault_Check/8(BSW_UdcDigitalValue)
  BSW_TempMotorDigitalValue/1 -> Circuit_Fault_Check/7(BSW_TempMotorDigitalValue)
  BSW_TempHSDigitalValue/1 -> Circuit_Fault_Check/6(BSW_TempHSDigitalValue)
  Circuit_Fault_Check/8(UdcCircuitFltInfo) -> UdcCircuitFltInfo/1
  Circuit_Fault_Check/6(TpcuCircuitFltInfo) -> TpcuCircuitFltInfo/1
  Circuit_Fault_Check/7(TmotorCircuitFltInfo) -> TmotorCircuitFltInfo/1
  CANBusFaultIn/1 -> CAN_Fault_Check/1(CANBusFaultIn)
  CAN_Fault_Check/1(CANFltInfo) -> CANFltInfo/1

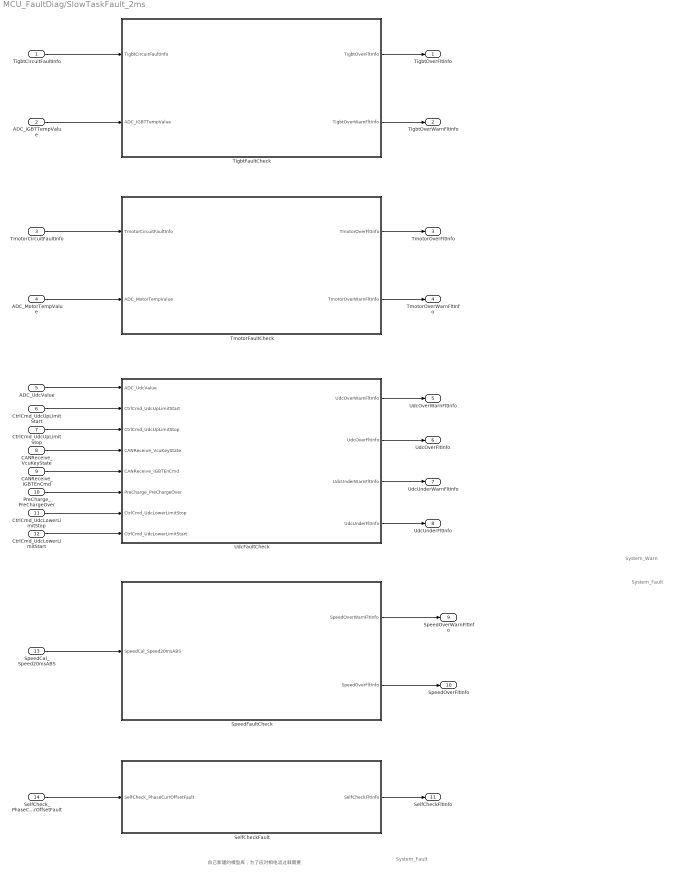
== system MCU_FaultDiag/SlowTaskFault_2ms ==
  note: System_Fault
  note: System_Warn
  note: System_Fault
  note: 自己新建的模型库，为了应对相电流过载需要
  TigbtCircuitFaultInfo : Inport
  ADC_IGBTTempValue : Inport  Port=2
  TmotorCircuitFaultInfo : Inport  Port=3
  ADC_MotorTempValue : Inport  Port=4
  ADC_UdcValue : Inport  Port=5
  CtrlCmd_UdcUpLimitStart : Inport  Port=6
  CtrlCmd_UdcUpLimitStop : Inport  Port=7
  CANReceive_VcuKeyState : Inport  Port=8
  CANReceive_IGBTEnCmd : Inport  Port=9
  PreCharge_PreChargeOver : Inport  Port=10
  CtrlCmd_UdcLowerLimitStop : Inport  Port=11
  CtrlCmd_UdcLowerLimitStart : Inport  Port=12
  SpeedCal_Speed20msABS : Inport  Port=13
  SelfCheck_PhaseCurrOffsetFault : Inport  Port=14
  SelfCheckFault : Subsystem
  SpeedFaultCheck : Subsystem
  TigbtFaultCheck : Subsystem  TreatAsAtomicUnit=on
      settings: RTWSystemCode=Nonreusable function
  TmotorFaultCheck : Subsystem  TreatAsAtomicUnit=on
      settings: RTWSystemCode=Nonreusable function
  UdcFaultCheck : Subsystem
  TigbtOverFltInfo : Outport
  TigbtOverWarnFltInfo : Outport  Port=2
  TmotorOverFltInfo : Outport  Port=3
  TmotorOverWarnFltInfo : Outport  Port=4
  UdcOverWarnFltInfo : Outport  Port=5
  UdcOverFltInfo : Outport  Port=6
  UdcUnderWarnFltInfo : Outport  Port=7
  UdcUnderFltInfo : Outport  Port=8
  SpeedOverWarnFltInfo : Outport  Port=9
  SpeedOverFltInfo : Outport  Port=10
  SelfCheckFltInfo : Outport  Port=11
  wires:
  TigbtCircuitFaultInfo/1 -> TigbtFaultCheck/1(TigbtCircuitFaultInfo)
  ADC_IGBTTempValue/1 -> TigbtFaultCheck/2(ADC_IGBTTempValue)
  TmotorCircuitFaultInfo/1 -> TmotorFaultCheck/1(TmotorCircuitFaultInfo)
  ADC_MotorTempValue/1 -> TmotorFaultCheck/2(ADC_MotorTempValue)
  TigbtFaultCheck/1(TigbtOverFltInfo) -> TigbtOverFltInfo/1
  TigbtFaultCheck/2(TigbtOverWarnFltInfo) -> TigbtOverWarnFltInfo/1
  TmotorFaultCheck/1(TmotorOverFltInfo) -> TmotorOverFltInfo/1
  TmotorFaultCheck/2(TmotorOverWarnFltInfo) -> TmotorOverWarnFltInfo/1
  CANReceive_VcuKeyState/1 -> UdcFaultCheck/4(CANReceive_VcuKeyState)
  CANReceive_IGBTEnCmd/1 -> UdcFaultCheck/5(CANReceive_IGBTEnCmd)
  ADC_UdcValue/1 -> UdcFaultCheck/1(ADC_UdcValue)
  PreCharge_PreChargeOver/1 -> UdcFaultCheck/6(PreCharge_PreChargeOver)
  CtrlCmd_UdcLowerLimitStop/1 -> UdcFaultCheck/7(CtrlCmd_UdcLowerLimitStop)
  CtrlCmd_UdcLowerLimitStart/1 -> UdcFaultCheck/8(CtrlCmd_UdcLowerLimitStart)
  CtrlCmd_UdcUpLimitStart/1 -> UdcFaultCheck/2(CtrlCmd_UdcUpLimitStart)
  CtrlCmd_UdcUpLimitStop/1 -> UdcFaultCheck/3(CtrlCmd_UdcUpLimitStop)
  UdcFaultCheck/1(UdcOverWarnFltInfo) -> UdcOverWarnFltInfo/1
  UdcFaultCheck/2(UdcOverFltInfo) -> UdcOverFltInfo/1
  UdcFaultCheck/3(UdcUnderWarnFltInfo) -> UdcUnderWarnFltInfo/1
  UdcFaultCheck/4(UdcUnderFltInfo) -> UdcUnderFltInfo/1
  SpeedCal_Speed20msABS/1 -> SpeedFaultCheck/1(SpeedCal_Speed20msABS)
  SpeedFaultCheck/1(SpeedOverWarnFltInfo) -> SpeedOverWarnFltInfo/1
  SpeedFaultCheck/2(SpeedOverFltInfo) -> SpeedOverFltInfo/1
  SelfCheck_PhaseCurrOffsetFault/1 -> SelfCheckFault/1(SelfCheck_PhaseCurrOffsetFault)
  SelfCheckFault/1(SelfCheckFltInfo) -> SelfCheckFltInfo/1

== system MCU_FaultDiag/FaultModeManage/Arbitration ==
  note: InterruptFault
      |
      | Ia_Instant_Fault
      | 1
      |
      | Ib_Instant_Fault
      | 1
      |
      | Ic_Instant_Fault
      | 1
      |
      | Speed_Instant_Fault
      |
      | Ace_Instant_Fault
  note: System_Fault
      |
      | TigbtOverFault
      | 1
      |
      | TmotorOverFault
      | 1
      |
      | UdcOverFault
      | 1
      |
      | UdcUnderFault
      | 1
      |
      | SpeedOverFault
      | 1
      |
      | TZFault
      | 1
      |
      | SelfCheckFlt
      | 1
  note: SystemWarn
      |
      | TigbtOverWarnFault
      |
      | TmotorOverWarnFault
      |
      | UdcOverWarnFault
      |
      | UdcUnderWarnFault
      |
      | SpeedOverWarnFault
      |
      | IaOverLoadFault
      |
      | IbOverLoadFault
      |
      | IcOverLoadFault
  note: DiagnoseFault
      |
      | TigbtCircuitFltInfo
      |
      | IdcCircuitFltInfo
      |
      | IaCircuitFltInfo
      |
      | IbCircuitFltInfo
      |
      | IcCircuitFltInfo
      |
      | TpcuCircuitFltInfo
      |
      | TmotorCircuitFltInfo
      |
      | UdcCircuitFltInfo
  WorkCmdSource_ModeCmd : Inport
  Interrupt_Fault : Inport  Port=2
  System_Fault : Inport  Port=3
  Diagnose_Fault : Inport  Port=4
  Compare To Constant : simulink/Logic and Bit Operations/Compare To Constant  relop===  const=cSingleBoardMode  OutDataTypeStr=boolean
  Compare To Constant1 : simulink/Logic and Bit Operations/Compare To Constant  relop===  const=cAgeingMode  OutDataTypeStr=boolean
  If : If  NumInputs=2  IfExpression=u1 == 1  ElseIfExpressions=u2 == 1
  If Action Subsystem : Subsystem  TreatAsAtomicUnit=on
  If Action Subsystem1 : Subsystem  TreatAsAtomicUnit=on
  If Action Subsystem2 : Subsystem  TreatAsAtomicUnit=on
  Merge : Merge  Inputs=3
  Merge1 : Merge  Inputs=3
  ClosePWMFlg : Outport
  TorqueZeroFlg : Outport  Port=2
  wires:
  WorkCmdSource_ModeCmd/1 -> Compare To Constant1/1, Compare To Constant/1
  Compare To Constant/1 -> If/1
  Compare To Constant1/1 -> If/2
  If/1 -> If Action Subsystem/Action
  Diagnose_Fault/1 -> If Action Subsystem2/3(Diagnose_Fault), If Action Subsystem1/3(Diagnose_Fault)
  System_Fault/1 -> If Action Subsystem2/2(System_Fault), If Action Subsystem1/2(System_Fault)
  Interrupt_Fault/1 -> If Action Subsystem2/1(Interrupt_Fault), If Action Subsystem1/1(Interrupt_Fault)
  If/2 -> If Action Subsystem1/Action
  If/3 -> If Action Subsystem2/Action
  If Action Subsystem/1(ClosePWMFlg) -> Merge/1
  If Action Subsystem1/1(ClosePWMFlg) -> Merge/2
  If Action Subsystem2/1(ClosePWMFlg) -> Merge/3
  If Action Subsystem/2(TorqueZeroFlg) -> Merge1/1
  If Action Subsystem1/2(TorqueZeroFlg) -> Merge1/2
  If Action Subsystem2/2(TorqueZeroFlg) -> Merge1/3
  Merge/1 -> ClosePWMFlg/1
  Merge1/1 -> TorqueZeroFlg/1

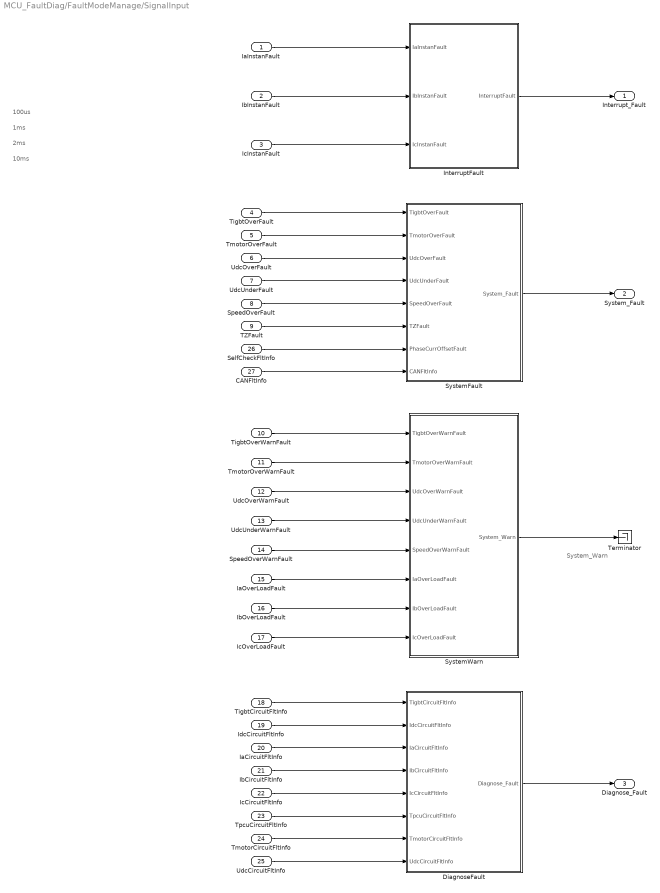
== system MCU_FaultDiag/FaultModeManage/SignalInput ==
  note: System_Warn
  note: 10ms
  note: 2ms
  note: 1ms
  note: 100us
  IaInstanFault : Inport
  IbInstanFault : Inport  Port=2
  IcInstanFault : Inport  Port=3
  TigbtOverFault : Inport  Port=4
  TmotorOverFault : Inport  Port=5
  UdcOverFault : Inport  Port=6
  UdcUnderFault : Inport  Port=7
  SpeedOverFault : Inport  Port=8
  TZFault : Inport  Port=9
  TigbtOverWarnFault : Inport  Port=10
  TmotorOverWarnFault : Inport  Port=11
  UdcOverWarnFault : Inport  Port=12
  UdcUnderWarnFault : Inport  Port=13
  SpeedOverWarnFault : Inport  Port=14
  IaOverLoadFault : Inport  Port=15
  IbOverLoadFault : Inport  Port=16
  IcOverLoadFault : Inport  Port=17
  TigbtCircuitFltInfo : Inport  Port=18
  IdcCircuitFltInfo : Inport  Port=19
  IaCircuitFltInfo : Inport  Port=20
  IbCircuitFltInfo : Inport  Port=21
  IcCircuitFltInfo : Inport  Port=22
  TpcuCircuitFltInfo : Inport  Port=23
  TmotorCircuitFltInfo : Inport  Port=24
  UdcCircuitFltInfo : Inport  Port=25
  SelfCheckFltInfo : Inport  Port=26
  CANFltInfo : Inport  Port=27
  DiagnoseFault : Subsystem
  InterruptFault : Subsystem
  SystemFault : Subsystem
  SystemWarn : Subsystem
  Terminator : Terminator
  Interrupt_Fault : Outport
  System_Fault : Outport  Port=2
  Diagnose_Fault : Outport  Port=3
  wires:
  SpeedOverFault/1 -> SystemFault/5(SpeedOverFault)
  UdcOverFault/1 -> SystemFault/3(UdcOverFault)
  TigbtOverWarnFault/1 -> SystemWarn/1(TigbtOverWarnFault)
  TmotorOverWarnFault/1 -> SystemWarn/2(TmotorOverWarnFault)
  IbInstanFault/1 -> InterruptFault/2(IbInstanFault)
  UdcUnderFault/1 -> SystemFault/4(UdcUnderFault)
  IcInstanFault/1 -> InterruptFault/3(IcInstanFault)
  SystemWarn/1(System_Warn) -> Terminator/1
  IaInstanFault/1 -> InterruptFault/1(IaInstanFault)
  TmotorOverFault/1 -> SystemFault/2(TmotorOverFault)
  TigbtOverFault/1 -> SystemFault/1(TigbtOverFault)
  IaOverLoadFault/1 -> SystemWarn/6(IaOverLoadFault)
  UdcUnderWarnFault/1 -> SystemWarn/4(UdcUnderWarnFault)
  SpeedOverWarnFault/1 -> SystemWarn/5(SpeedOverWarnFault)
  IcOverLoadFault/1 -> SystemWarn/8(IcOverLoadFault)
  IbOverLoadFault/1 -> SystemWarn/7(IbOverLoadFault)
  UdcOverWarnFault/1 -> SystemWarn/3(UdcOverWarnFault)
  InterruptFault/1(InterruptFault) -> Interrupt_Fault/1
  SystemFault/1(System_Fault) -> System_Fault/1
  TZFault/1 -> SystemFault/6(TZFault)
  DiagnoseFault/1(Diagnose_Fault) -> Diagnose_Fault/1
  TigbtCircuitFltInfo/1 -> DiagnoseFault/1(TigbtCircuitFltInfo)
  IdcCircuitFltInfo/1 -> DiagnoseFault/2(IdcCircuitFltInfo)
  IaCircuitFltInfo/1 -> DiagnoseFault/3(IaCircuitFltInfo)
  IbCircuitFltInfo/1 -> DiagnoseFault/4(IbCircuitFltInfo)
  IcCircuitFltInfo/1 -> DiagnoseFault/5(IcCircuitFltInfo)
  TpcuCircuitFltInfo/1 -> DiagnoseFault/6(TpcuCircuitFltInfo)
  TmotorCircuitFltInfo/1 -> DiagnoseFault/7(TmotorCircuitFltInfo)
  UdcCircuitFltInfo/1 -> DiagnoseFault/8(UdcCircuitFltInfo)
  SelfCheckFltInfo/1 -> SystemFault/7(PhaseCurrOffsetFault)
  CANFltInfo/1 -> SystemFault/8(CANFltInfo)

== system MCU_FaultDiag/HighTaskFault_100us/InterruptFaultCheck_100us ==
  FOC_IaValue : Inport
  FOC_IbValue : Inport  Port=2
  FOC_IcValue : Inport  Port=3
  SelfCheck_SelfCheckOverFlg : Inport  Port=4
  InstantFaultOfIa : Subsystem  TreatAsAtomicUnit=on
      settings: RTWSystemCode=Nonreusable function
  InstantFaultOfIb : Subsystem  TreatAsAtomicUnit=on
      settings: RTWSystemCode=Nonreusable function
  InstantFaultOfIc : Subsystem  TreatAsAtomicUnit=on
      settings: RTWSystemCode=Nonreusable function
  TZFaultGet_100us : Subsystem  TreatAsAtomicUnit=on
      settings: RTWSystemCode=Nonreusable function
  IaInstantFltInfo : Outport
  IbInstantFltInfo : Outport  Port=2
  IcInstantFltInfo : Outport  Port=3
  TZFltInfo : Outport  Port=4
  wires:
  FOC_IaValue/1 -> InstantFaultOfIa/1(IaValue)
  InstantFaultOfIa/1(IaInstantFltInfo) -> IaInstantFltInfo/1
  FOC_IbValue/1 -> InstantFaultOfIb/1(IbValue)
  InstantFaultOfIb/1(IbInstantFltInfo) -> IbInstantFltInfo/1
  FOC_IcValue/1 -> InstantFaultOfIc/1(IcValue)
  InstantFaultOfIc/1(IcInstantFltInfo) -> IcInstantFltInfo/1
  SelfCheck_SelfCheckOverFlg/1 -> TZFaultGet_100us/1(SelfCheck_SelfCheckOverFlg)
  TZFaultGet_100us/1(TZFltInfo) -> TZFltInfo/1

== system MCU_FaultDiag/MiddleTaskFault_1ms/PhaseFaultCheck ==
  ADC_IaValue : Inport
  SelfCheckFltInfo : Inport  Port=2
  ADC_IbValue : Inport  Port=3
  ADC_IcValue : Inport  Port=4
  TorqueCtrl_TorqueCmdFilter : Inport  Port=5
  Bus Selector : BusSelector  OutputSignals=SelfCheckFaultFlg
  IaOverLoadFaultCheck : Subsystem
  IbOverLoadFaultCheck : Subsystem
  IcOverLoadFaultCheck : Subsystem
  IaOverLoadFltInfo : Outport
  IbOverLoadFltInfo : Outport  Port=2
  IcOverLoadFltInfo : Outport  Port=3
  wires:
  ADC_IaValue/1 -> IaOverLoadFaultCheck/1(ADC_IaValue)
  IaOverLoadFaultCheck/1(IaOverLoadFltInfo) -> IaOverLoadFltInfo/1
  TorqueCtrl_TorqueCmdFilter/1 -> IcOverLoadFaultCheck/2(TorqueCtrl_TorqueCmdFilter), IbOverLoadFaultCheck/2(TorqueCtrl_TorqueCmdFilter), IaOverLoadFaultCheck/2(TorqueCtrl_TorqueCmdFilter)
  IbOverLoadFaultCheck/1(IbOverLoadFltInfo) -> IbOverLoadFltInfo/1
  ADC_IbValue/1 -> IbOverLoadFaultCheck/1(ADC_IbValue)
  ADC_IcValue/1 -> IcOverLoadFaultCheck/1(ADC_IcValue)
  IcOverLoadFaultCheck/1(IcOverLoadFltInfo) -> IcOverLoadFltInfo/1
  Bus Selector/1 -> IcOverLoadFaultCheck/3(PhaseCurrOffsetFault), IbOverLoadFaultCheck/3(SelfCheck_PhaseCurrOffsetFault), IaOverLoadFaultCheck/3(PhaseCurrOffsetFault)  "<SelfCheckFaultFlg>"
  SelfCheckFltInfo/1 -> Bus Selector/1

== system MCU_FaultDiag/SlowTaskFault_10ms/CAN_Fault_Check ==
  CANBusFaultIn : Inport
  Diag : Subsystem
  Params : Subsystem
  CANFltInfo : Outport
  wires:
  CANBusFaultIn/1 -> Diag/2(CANBusFaultIn)
  Params/1(CANFltParams) -> Diag/1(Params)
  Diag/1(CANFltInfo) -> CANFltInfo/1
